simulink model "QPSK_Rayleigh_SIMO_MRC"  (R2019b)
settings: Solver=VariableStepAuto  StartTime=0.0  StopTime=0.1  RelTol=1e-3
libraries: commchan3 x2, commdigbbndpm3 x2, commrandsrc3 x1, commsink2 x1
settings Model: Creator=Nikhil  LastModifiedBy=Nikhil

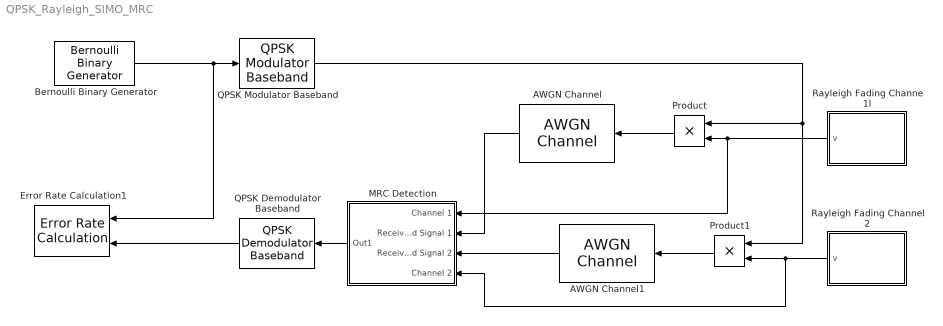
== system QPSK_Rayleigh_SIMO_MRC ==
  AWGN Channel : commchan3/AWGN Channel  InputProcessing=Columns as channels (frame based)  seed=12  noiseMode="Signal to noise ratio  (SNR)"  EbNodB=10  EsNodB=10  SNRdB=s  bitsPerSym=1  Ps=1  Tsym=1  variance=1
      settings: SourceProductName=Communications Toolbox
  AWGN Channel1 : commchan3/AWGN Channel  InputProcessing=Columns as channels (frame based)  seed=16  noiseMode="Signal to noise ratio  (SNR)"  EbNodB=10  EsNodB=10  SNRdB=s  bitsPerSym=1  Ps=1  Tsym=1  variance=1
      settings: SourceProductName=Communications Toolbox
  Bernoulli Binary Generator : commrandsrc3/Bernoulli Binary Generator  ProbabilityOfZero=0.5  SeedSource=Parameter  Seed=322  SampleTime=1e-6  SamplesPerFrame=2  OutputDataType=uint8  SimulateUsing=Interpreted execution
      settings: SourceProductName=Communications Toolbox
  Error Rate Calculation1 : commsink2/Error Rate Calculation  N=0  st_delay=0  cp_mode=Entire frame  subframe=[]  PMode=Workspace  WsName=Error_MRC  RsMode2=off  stop=off  numErr=100  maxBits=1e6
      settings: SourceProductName=Communications Toolbox
  MRC Detection : Subsystem
  Product : Product
  Product1 : Product
  QPSK Demodulator Baseband : commdigbbndpm3/QPSK Demodulator Baseband  OutType=Integer  DecType=Hard decision  VarSource=Dialog  Variance=1  Dec=Gray  Ph=pi/4  outDtype1=Inherit via internal rule  outDtype2=Inherit via internal rule  derotateFactorWordLen=16  derotateFactorDataTypeStr=Inherit: Same word length as input  derotateFactorLastDataTypeStr=Inherit: Same word length as input
      settings: SourceProductName=Communications Toolbox
  QPSK Modulator Baseband : commdigbbndpm3/QPSK Modulator Baseband  InType=Integer  Enc=Gray  Ph=pi/4  outDtype=Inherit via back propagation  outWordLen=16  outUDDataType=sfix(16)  outFracLenMode=Best precision  outFracLen=15  outDataTypeStr=Inherit: Inherit via back propagation  outLastDataTypeStr=Inherit: Inherit via back propagation
      settings: SourceProductName=Communications Toolbox
  Rayleigh Fading Channe 1l : Subsystem
  Rayleigh Fading Channel 2 : Subsystem
  wires:
  Bernoulli Binary Generator/1 -> QPSK Modulator Baseband/1, Error Rate Calculation1/1
  Product/1 -> AWGN Channel/1
  Rayleigh Fading Channe 1l/1(v) -> MRC Detection/1(Channel 1), Product/2
  QPSK Demodulator Baseband/1 -> Error Rate Calculation1/2
  Product1/1 -> AWGN Channel1/1
  Rayleigh Fading Channel 2/1(v) -> MRC Detection/4(Channel 2), Product1/2
  QPSK Modulator Baseband/1 -> Product1/1, Product/1
  MRC Detection/1(Out1) -> QPSK Demodulator Baseband/1
  AWGN Channel/1 -> MRC Detection/2(Received Signal 1)
  AWGN Channel1/1 -> MRC Detection/3(Received Signal 2)

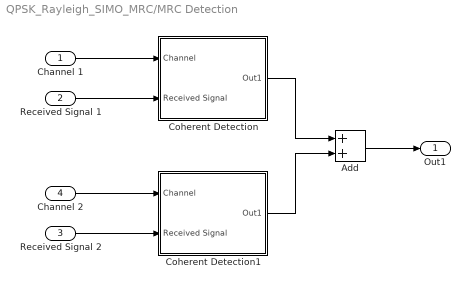
== system QPSK_Rayleigh_SIMO_MRC/MRC Detection ==
  Channel 1 : Inport
  Received Signal 1 : Inport  Port=2
  Received Signal 2 : Inport  Port=3
  Channel 2 : Inport  Port=4
  Add : Sum
  Coherent Detection : Subsystem
  Coherent Detection1 : Subsystem
  Out1 : Outport
  wires:
  Channel 1/1 -> Coherent Detection/1(Channel)
  Channel 2/1 -> Coherent Detection1/1(Channel)
  Received Signal 2/1 -> Coherent Detection1/2(Received Signal)
  Received Signal 1/1 -> Coherent Detection/2(Received Signal)
  Add/1 -> Out1/1
  Coherent Detection/1(Out1) -> Add/1
  Coherent Detection1/1(Out1) -> Add/2

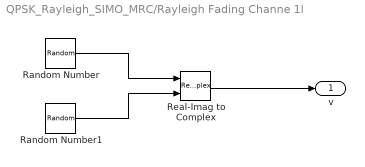
== system QPSK_Rayleigh_SIMO_MRC/Rayleigh Fading Channe 1l ==
  Random Number : RandomNumber  Variance=1/2  Seed=22  SampleTime=1e-6
  Random Number1 : RandomNumber  Variance=1/2  Seed=31  SampleTime=1e-6
  Real-Imag to Complex : RealImagToComplex
  v : Outport
  wires:
  Real-Imag to Complex/1 -> v/1
  Random Number/1 -> Real-Imag to Complex/1
  Random Number1/1 -> Real-Imag to Complex/2

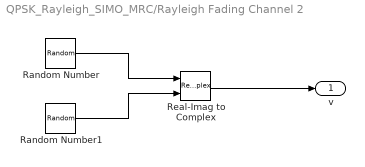
== system QPSK_Rayleigh_SIMO_MRC/Rayleigh Fading Channel 2 ==
  Random Number : RandomNumber  Variance=1/2  Seed=420  SampleTime=1e-6
  Random Number1 : RandomNumber  Variance=1/2  Seed=69  SampleTime=1e-6
  Real-Imag to Complex : RealImagToComplex
  v : Outport
  wires:
  Real-Imag to Complex/1 -> v/1
  Random Number/1 -> Real-Imag to Complex/1
  Random Number1/1 -> Real-Imag to Complex/2

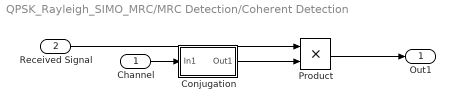
== system QPSK_Rayleigh_SIMO_MRC/MRC Detection/Coherent Detection ==
  Channel : Inport
  Received Signal : Inport  Port=2
  Conjugation : Subsystem
  Product : Product
  Out1 : Outport
  wires:
  Channel/1 -> Conjugation/1(In1)
  Product/1 -> Out1/1
  Received Signal/1 -> Product/1
  Conjugation/1(Out1) -> Product/2

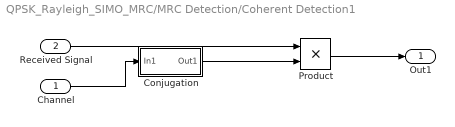
== system QPSK_Rayleigh_SIMO_MRC/MRC Detection/Coherent Detection1 ==
  Channel : Inport
  Received Signal : Inport  Port=2
  Conjugation : Subsystem
  Product : Product
  Out1 : Outport
  wires:
  Channel/1 -> Conjugation/1(In1)
  Product/1 -> Out1/1
  Received Signal/1 -> Product/1
  Conjugation/1(Out1) -> Product/2

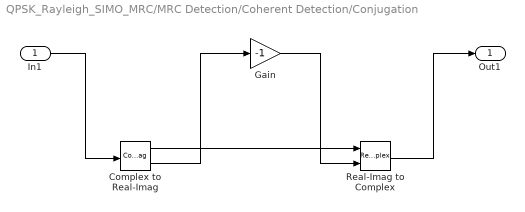
== system QPSK_Rayleigh_SIMO_MRC/MRC Detection/Coherent Detection/Conjugation ==
  In1 : Inport
  Complex to Real-Imag : ComplexToRealImag
  Gain : Gain  Gain=-1
  Real-Imag to Complex : RealImagToComplex
  Out1 : Outport
  wires:
  In1/1 -> Complex to Real-Imag/1
  Complex to Real-Imag/1 -> Real-Imag to Complex/1
  Complex to Real-Imag/2 -> Gain/1
  Gain/1 -> Real-Imag to Complex/2
  Real-Imag to Complex/1 -> Out1/1

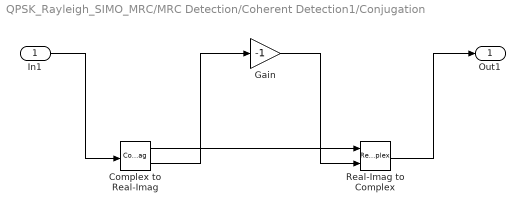
== system QPSK_Rayleigh_SIMO_MRC/MRC Detection/Coherent Detection1/Conjugation ==
  In1 : Inport
  Complex to Real-Imag : ComplexToRealImag
  Gain : Gain  Gain=-1
  Real-Imag to Complex : RealImagToComplex
  Out1 : Outport
  wires:
  In1/1 -> Complex to Real-Imag/1
  Complex to Real-Imag/1 -> Real-Imag to Complex/1
  Complex to Real-Imag/2 -> Gain/1
  Gain/1 -> Real-Imag to Complex/2
  Real-Imag to Complex/1 -> Out1/1
